simulink model "Complete_Model_Control"  (R2018a)
settings: Solver=VariableStepAuto  StartTime=0.0  StopTime=40  RelTol=1e-3
values from neighbouring files (symbols this model uses):
  A_ad = [zeros(3,3), eye(3) ... (first row only)    [Admittance.m]
  Ak = zeros(18,18)    [Kalman_filter.m]
  B_ad = [zeros(3,3), zeros(3,3) ... (first row only)    [Admittance.m]
  Bk = zeros(18,4)    [Kalman_filter.m]
  C_ad = [eye(3), zeros(3,3)]    [Admittance.m]
  Ck = zeros(6,18)    [Kalman_filter.m]
  D_ad = zeros(3,6)    [Admittance.m]
  Dk = zeros(6,4)    [Kalman_filter.m]
  p = menu('Choose the problem: 1 for trajectory tracking and 2 for regulation', 1,2)    [Admittance.m]
  par = [m;m1;Ix;Iy;Iz;Ir;Om_r;d;l;g;T1;T2]    [Quadrotor_Model.m]
  Tn = 0.001    [Kalman_filter.m]
  V = 10*eye(6)    [Kalman_filter.m]
  v = 0.001*ones(6,1)    [Kalman_filter.m]
undefined symbols (not defined in the file or in its folder): Continuous, Time
libraries: ctrlSharedLib x1
settings Model: Creator=Pimentel  LastModifiedBy=Pimentel

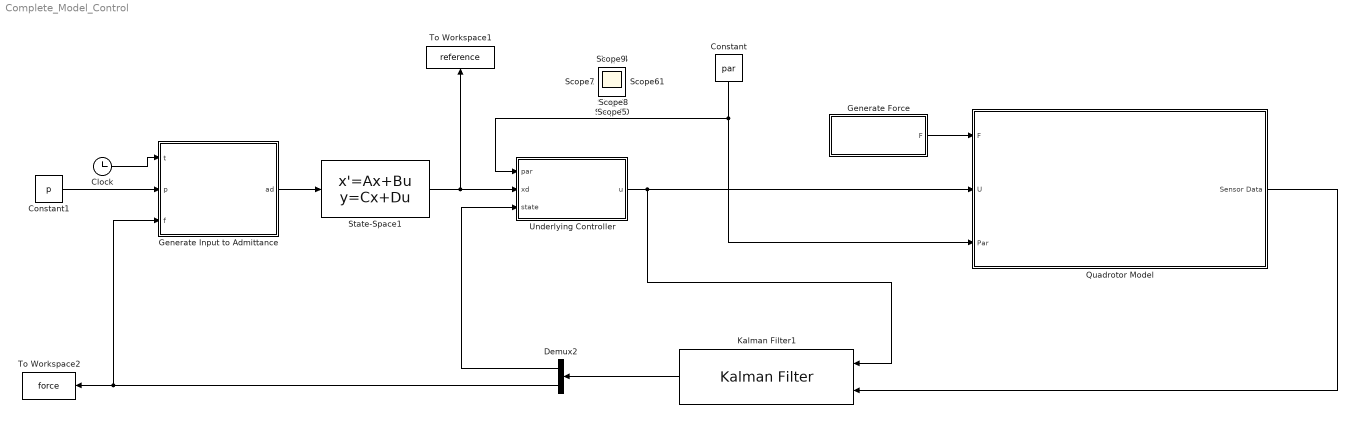
== system Complete_Model_Control ==
  Clock : Clock
  Constant : Constant  Value=par
  Constant1 : Constant  Value=p
  Demux2 : Demux  Outputs=[15, 3]
  Generate Force : Subsystem
  "Generate Input to Admittance " : MATLAB Function  TreatAsAtomicUnit=on
  Kalman Filter1 : ctrlSharedLib/Kalman Filter  TimeDomain=Continuous-Time  UseCurrentEstimator=on  ModelSource=Individual A, B, C, D matrices  ModelSourceVariable=ss(0.95,1,1,0,1)  A=Ak  B=Bk  C=Ck  D=Dk  NumberOfStates=1  NumberOfInputs=1  NumberOfOutputs=1  InitialEstimateSource=Dialog  X0=0  P0=10  UseK=off  UseGH=off  NumberOfProcessNoiseInputs=1  G=1  TimeInvariantG=on  H=0  TimeInvariantH=on  Q=W  TimeInvariantQ=on  R=V  TimeInvariantR=on  N=0  TimeInvariantN=on  AddInputPort=on  AddEnablePort=off  OutputEstimatedY=off  OutputP=off  Ts=-1
      settings: SourceProductBaseCode=CT
  Quadrotor Model : Subsystem
  State-Space1 : StateSpace  A=A_ad  B=B_ad  C=C_ad  D=D_ad  InitialCondition=[0 0 0 0 0 0]
  To Workspace1 : ToWorkspace  VariableName=reference  SaveFormat=Structure With Time  SampleTime=-1
  To Workspace2 : ToWorkspace  VariableName=force  SaveFormat=Structure With Time  SampleTime=-1
  Underlying Controller : MATLAB Function  TreatAsAtomicUnit=on
  Scope{,1..11} (12 alike) : Scope
  wires:
  Underlying Controller/1(u) -> Kalman Filter1/1, Quadrotor Model/2("U ")
  Clock/1 -> "Generate Input to Admittance "/1(t)
  Constant/1 -> Quadrotor Model/3("Par "), Underlying Controller/1(par)
  State-Space1/1 -> Underlying Controller/2(xd), To Workspace1/1
  Demux2/1 -> Underlying Controller/3(state)
  Demux2/2 -> To Workspace2/1, "Generate Input to Admittance "/3(f)
  Kalman Filter1/1 -> Demux2/1
  "Generate Input to Admittance "/1(ad) -> State-Space1/1
  Generate Force/1(F) -> Quadrotor Model/1(F)
  Quadrotor Model/1(Sensor Data) -> Kalman Filter1/2
  Constant1/1 -> "Generate Input to Admittance "/2(p)

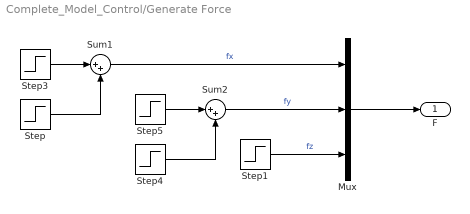
== system Complete_Model_Control/Generate Force ==
  Mux : Mux  Inputs=3
  Step : Step  Time=6  After=-3  SampleTime=0
  Step1 : Step  After=0  SampleTime=0
  Step3 : Step  After=3  SampleTime=0
  Step4 : Step  Time=6  After=-1  SampleTime=0
  Step5 : Step  SampleTime=0
  Sum1 : Sum  Inputs=|++
  Sum2 : Sum  Inputs=|++
  F : Outport
  wires:
  Mux/1 -> F/1
  Sum1/1 -> Mux/1  "fx"
  Step/1 -> Sum1/2
  Step1/1 -> Mux/3  "fz"
  Step3/1 -> Sum1/1
  Step4/1 -> Sum2/2
  Step5/1 -> Sum2/1
  Sum2/1 -> Mux/2  "fy"

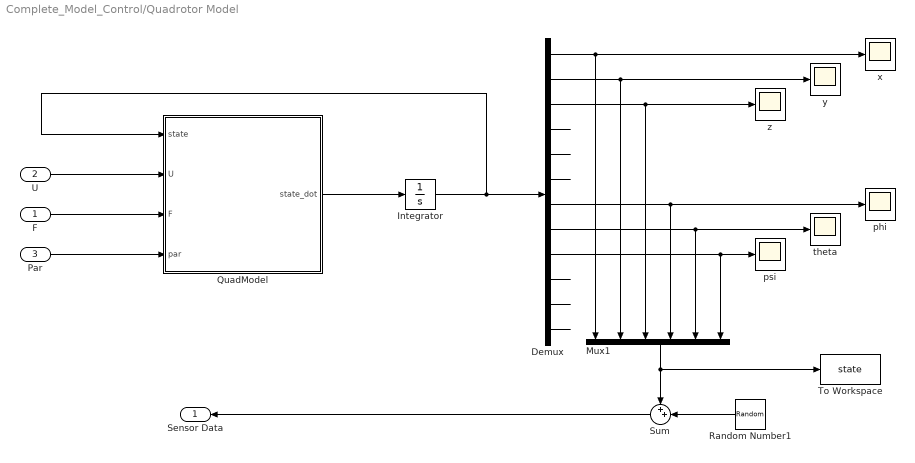
== system Complete_Model_Control/Quadrotor Model ==
  F : Inport
  "U " : Inport  Port=2
  "Par " : Inport  Port=3
  Demux : Demux  Outputs=12
  Integrator : Integrator  InitialCondition=[0 0 0 0 0 0 0 0 0 0 0 0]
  Mux1 : Mux  Inputs=6
  QuadModel : MATLAB Function  TreatAsAtomicUnit=on
  Random Number1 : RandomNumber  Mean=[0 0 0 0 0 0]  Variance=v  SampleTime=Tn
  Sum : Sum  Inputs=++|
  To Workspace : ToWorkspace  VariableName=state  SaveFormat=Structure With Time  SampleTime=-1
  phi : Scope
  psi : Scope
  theta : Scope
  "x " : Scope
  y : Scope
  z : Scope
  Sensor Data : Outport
  wires:
  Demux/11 -> ?
  Demux/4 -> ?
  Demux/10 -> ?
  "U "/1 -> QuadModel/2(U)
  Demux/12 -> ?
  Demux/7 -> Mux1/4, phi/1
  Mux1/1 -> To Workspace/1, Sum/1
  Integrator/1 -> QuadModel/1(state), Demux/1
  Demux/5 -> ?
  F/1 -> QuadModel/3(F)
  "Par "/1 -> QuadModel/4(par)
  Demux/1 -> Mux1/1, "x "/1
  Demux/9 -> Mux1/6, psi/1
  Demux/8 -> Mux1/5, theta/1
  Demux/3 -> Mux1/3, z/1
  Demux/6 -> ?
  Sum/1 -> Sensor Data/1
  QuadModel/1(state_dot) -> Integrator/1
  Random Number1/1 -> Sum/2
  Demux/2 -> Mux1/2, y/1

== matlab function Complete_Model_Control/Generate Input to Admittance  ==
  data: t input; p input; f input; ad output
function ad = generate(t,p,f)

if p == 1
    x_d = cos(t);
    y_d = sin(t);
    z_d = 0;
else
    x_d = 0;
    y_d = 0;
    z_d = 0;
end 

if f(1)>0.3
    fx = f(1);
else 
    fx = 0;
end

if f(2)>0.3
    fy = f(2);
else 
    fy = 0;
end

if f(3)>0.3
    fz = f(3);
else 
    fz = 0;    
end

ad = [x_d, y_d, z_d, fx, fy, fz]';

== matlab function Complete_Model_Control/Underlying Controller ==
  data: par input; xd input; state input; u output
function u = Pos_Att_Control(par, xd, state)

% Model Parameters 

m = par(1);
m1 = par(2);
Ix = par(3);
Iy = par(4);
Iz = par(5);
Ir = par(6);
Om_r = par(7);
d = par(8);
l = par(9);
g = par(10);

% State

x = state(1);
y = state(2);
z = state(3);
vx = state(4);
vy = state(5);
vz = state(6);
phi = state(7);
theta = state(8);
psi = state(9);
phi_dot = state(10);
theta_dot = state(11);
psi_dot = state(12);
tau_phi = state(13);
tau_theta = state(14);
tau_psi = state(15);

% Controller Gains 

kx_p = 20;
kx_d = 10;

ky_p = 20;
ky_d = 10;

kz_p = 2;
kz_d = 1;

k_phi = 20;
k_theta = 20;
k_psi = 1;

% Regulation task

x_d = xd(1);
y_d = xd(2);
z_d = xd(3);

vx_d = 0;
vy_d = 0;
vz_d = 0;

% Altitude Control

T_Tilde = m*(g-kz_p*(z_d - z) - kz_d*(vz_d - vz));
T = T_Tilde/m - g;

% Attitude Control

theta_d = -1/g*(kx_p*(x_d - x) + kx_d*(vx_d - vx));
phi_d = 1/g*(ky_p*(y_d - y) + ky_d*(vy_d - vy));
psi_d = 0;

phi_dot_cmd = k_phi*(phi_d - phi);
theta_dot_cmd = k_theta*(theta_d - theta);
psi_dot_cmd = k_psi*(psi_d - psi);

u = [T, phi_dot_cmd, theta_dot_cmd, psi_dot_cmd]';

== matlab function Complete_Model_Control/Quadrotor Model/QuadModel ==
  data: state input; U input; F input; state_dot output; par input
function state_dot = quadrotor_model(state,U,F,par)

% Model parameters

m=par(1);
m1=par(2);
Ix=par(3);
Iy=par(4);
Iz=par(5);
Ir=par(6);
Om_r=par(7);
d=par(8);
l=par(9);
g=par(10);
T1 = par(11);
T2 = par(12);

% Position
x=state(1);
y=state(2);
z=state(3);

vx=state(4);
vy=state(5);
vz=state(6);

% Attitude
phi=state(7);
theta=state(8);
psi=state(9);

dphi=state(10);
dtheta=state(11);
dpsi=state(12);

% Control Inputs

phi_dot_command = U(2);
theta_dot_command = U(3);
psi_dot_command = U(4);

tau_phi = Ix/T2*(phi_dot_command - dphi);
tau_theta = Iy/T2*(theta_dot_command - dtheta);
tau_psi = Iz/T2*(psi_dot_command - dpsi);
T = (U(1) + g)*m;

f_x = F(1);
f_y = F(2);
f_z = F(3);

% Dynamics

xdot=vx;
vxdot = -(T/m)*(cos(phi)*sin(theta)*cos(psi)+sin(phi)*sin(psi)) + f_x/m;

ydot=vy;
vydot = -(T/m)*(cos(phi)*sin(theta)*sin(psi)-sin(phi)*cos(psi)) + f_y/m;

zdot=vz;
vzdot = -(- g + (T/m)*(cos(phi)*cos(theta))) + f_z/m;

phidot=dphi;
dphidot =  ((Iy-Iz)/Ix)*dtheta*dpsi + (Ir/Ix)*dtheta*Om_r +(l/Ix)*tau_phi;

thetadot=dtheta;
dthetadot = ((Iz-Ix)/Iy)*dphi*dpsi - (Ir/Iy)*dphi*Om_r +(l/Iy)*tau_theta;

psidot=dpsi;
dpsidot =  ((Ix-Iy)/Iz)*dphi*dtheta + (1/Iz)*tau_psi;

state_dot = [xdot, ydot, zdot, vxdot, vydot, vzdot, phidot, thetadot, psidot, dphidot, dthetadot, dpsidot]';
